simulink model "frac_test_caojx"  (Simulink 8.3)
settings: Solver=ode45  StartTime=0.0  StopTime=10.0  RelTol=1e-3
values from neighbouring files (symbols this model uses):
  FraOrder = CalFracPra( FraAlpha,n)    [initialization1.m]    (also in test_ousta_fod.m = CalFracPra(-0.5,4))
settings Model: Creator=wayne  LastModifiedBy=wayne
settings DataIOCC: SignalLoggingSaveFormat=Dataset
settings DebuggingCC: UnderspecifiedInitializationDetection=Simplified  StateNameClashWarn=none
settings GRTTargetCC: CombineOutputUpdateFcns=on  GRTInterface=off

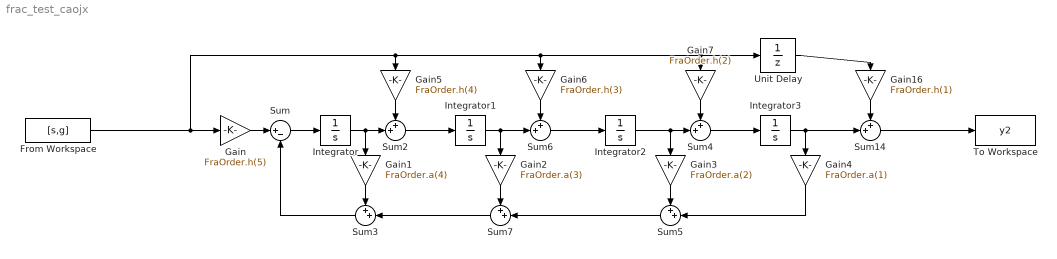
== system frac_test_caojx ==
  From Workspace : FromWorkspace  VariableName=[s,g]  SampleTime=0
  Gain : Gain  Gain=FraOrder.h(5)
  Gain1 : Gain  Gain=FraOrder.a(4)
  Gain16 : Gain  Gain=FraOrder.h(1)
  Gain2 : Gain  Gain=FraOrder.a(3)
  Gain3 : Gain  Gain=FraOrder.a(2)
  Gain4 : Gain  Gain=FraOrder.a(1)
  Gain5 : Gain  Gain=FraOrder.h(4)
  Gain6 : Gain  Gain=FraOrder.h(3)
  Gain7 : Gain  Gain=FraOrder.h(2)
  Integrator{,1..3} (4 alike) : Integrator
  Sum : Sum  Inputs=|+-
  Sum{2..7,14} (7 alike) : Sum  Inputs=++|
  To Workspace : ToWorkspace  VariableName=y2  SaveFormat=Structure With Time  SampleTime=-1
  Unit Delay : UnitDelay  SampleTime=-1
  wires:
  Sum/1 -> Integrator/1
  Integrator/1 -> Sum2/2, Gain1/1
  Sum2/1 -> Integrator1/1
  Integrator1/1 -> Gain2/1, Sum6/2
  Sum3/1 -> Sum/2
  Gain/1 -> Sum/1
  Gain1/1 -> Sum3/1
  Integrator2/1 -> Sum4/2, Gain3/1
  Sum4/1 -> Integrator3/1
  Integrator3/1 -> Gain4/1, Sum14/2
  Sum5/1 -> Sum7/2
  Gain3/1 -> Sum5/1
  Gain4/1 -> Sum5/2
  Sum6/1 -> Integrator2/1
  Gain5/1 -> Sum2/1
  Gain6/1 -> Sum6/1
  Gain7/1 -> Sum4/1
  Sum7/1 -> Sum3/2
  Gain2/1 -> Sum7/1
  From Workspace/1 -> Gain/1, Gain5/1, Gain6/1, Gain7/1, Unit Delay/1
  Gain16/1 -> Sum14/1
  Sum14/1 -> To Workspace/1
  Unit Delay/1 -> Gain16/1
